simulink model "combinedTxRx_ADIDMA"  (R2017b)
settings: Solver=FixedStepDiscrete  StartTime=0.0  StopTime=10.0  RelTol=1e-3
InitFcn:
  | numHeaderBits = 16;
  | %numPreambleBits = 250;
  | AGCBarkerSymbols = 160+28;
  | EQTrainingSymbols = 250;
  | CRCGeneratorLag = 34; % CRCLen + 2
  | 
  | %% AGC Preamble
  | B13bipolar = [0 0 0 0 0 2 2 0 0 2 0 2];
  | rep = [B13bipolar, B13bipolar(1:4)];
  | AGCBarker = repmat(rep,1,10);
  | % Second preamble part
  | B11bipolar = [0 0 0 2 2 2 0 2  2 0 2];
  | TimingBarker = [B11bipolar,B11bipolar,B11bipolar,B11bipolar(1:6)];
  | PreambleBarkersInts = [AGCBarker, TimingBarker];
  | % Convert integer into their bit representation
  | PreambleBarkersBits = zeros(1,length(PreambleBarkersInts)*2);
  | PreambleBarkersBits(1:2:end) = (PreambleBarkersInts==2);
  | 
  | % Constants
  | % First preamble part
  | B13bipolar = [0 0 0 0 0 2 2 0 0 2 0 2];
  | rep = [B13bipolar, B13bipolar(1:4)];
  | AGCBarker = repmat(rep,1,10);
  | % Second preamble part
  | B11bipolar = [0 0 0 2 2 2 0 2  2 0 2];
  | TimingBarker = [B11bipolar,B11bipolar,B11bipolar(1:6)];
  | PreambleBarkersInts = [AGCBarker, TimingBarker];
  | % Convert integer into their bit representation
  | PreambleBarkersBits = false(1,length(PreambleBarkersInts)*2);
  | PreambleBarkersBits(1:2:end) = logical(PreambleBarkersInts==2);
  | pLen = uint16(length(PreambleBarkersBits));
  | 
  | 
  | %%%%%%%%%%%%%%%%%%%%%%%%%%
  | %% RX
  | %%%%%%%%%%%%%%%%%%%%%%%%%%
  | 
  | barker = comm.BarkerCode('SamplesPerFrame', 28, 'Length', 11);
  | seq = barker()+1;
  | M = 4;
  | hPSKModTrain   = comm.PSKModulator(M, ...
  |     'PhaseOffset',pi/4, ...
  |     'SymbolMapping','Binary');
  | xPreambleSeq = hPSKModTrain(seq);
  | 
  | 
  | %%%%%%%%%%%%
  | 
  | % AGC Preamble
  | reps = 5;
  | barker = comm.BarkerCode('SamplesPerFrame', 16, 'Length', 13);
  | seq = barker()+1;
  | %preamble = zeros(16*reps,1);
  | preambleFull = repmat(seq,reps,1);
  | rctFilt = comm.RaisedCosineTransmitFilter('FilterSpanInSymbols', 128,...
  | 'RolloffFactor',0.5,...
  | 'OutputSamplesPerSymbol',4);
  | preambleFullFilt = rctFilt(preambleFull);
  | 
  | %%%%%%%%%%%%
  | 
  | RadioSampleRate = 1e6;
  | %RadioSampleRate = 20e6;
  | RadioFrameLength = 1e5;
  | 
  | VibertiTracebackLength = 34+20;
  | numTrainingSamples = 250;
  | crc32Poly = [1 0 0 0 0 0 1 0 0 1 1 0 0 0 0 0 1 0 0 0 1 1 1 0 1 1 0 1 1 0 1 1 1];
  | crcDecodeLag = length(crc32Poly)-1+2;
  | 
  | %%%%%%%%%%%%
  | 
  | beta = 0.5;
  | span = 8;
  | sps = 4;
  | filterGain = 1;
  | coeff = rcosdesign(beta, span, sps, 'sqrt')*filterGain;
  | 
  | %%%%%%%%%%%%
  | 
  | samplesPerSymbol = 4;
  | maxPacketBits = 8*1500;
  | bItsPerSymbol = 2;
  | CodeRate = 2;
  | tailSymbols = 40;
  | maxPayloadSymbols = maxPacketBits*CodeRate/bItsPerSymbol+tailSymbols;
  | 
  | 
  | %%%%%%%%%%%%
  | 
  | NormalizedLoopBandwidths = 0.01:0.01:0.4;
  | K1 = zeros(length(NormalizedLoopBandwidths),1);
  | K2 = zeros(length(NormalizedLoopBandwidths),1);
  | 
  | for index=1:length(NormalizedLoopBandwidths)
  |     DampingFactor = 4*1/sqrt(2);
  |     samplesPerSymbolFR = 1;
  |     NormalizedLoopBandwidth = NormalizedLoopBandwidths(index);
  | 
  |     %%
  |     PhaseRecoveryLoopBandwidth = NormalizedLoopBandwidth*samplesPerSymbolFR;
  | 
  |     PhaseRecoveryGain = samplesPerSymbolFR;
  | 
  |     PhaseErrorDetectorGain = 1;
  | 
  |     %%
  |     theta = PhaseRecoveryLoopBandwidth/...
  |         ((DampingFactor + 0.25/DampingFactor)*samplesPerSymbolFR);
  | 
  |     d = 1 + 2*DampingFactor*theta + theta*theta;
  | 
  |     % K1
  |     K1(index) = (4*DampingFactor*theta/d)/...
  |         (PhaseErrorDetectorGain*PhaseRecoveryGain);
  |     % K2
  |     K2(index) = (4/samplesPerSymbol*theta*theta/d)/...
  |         (PhaseErrorDetectorGain*PhaseRecoveryGain);
  | 
  | end
  | K1 = fi(K1,0);
  | K2 = fi(K2,0);
undefined symbols (not defined in the file or in its folder): j
libraries: simulink x20, dsphdlfiltering x20, hdlsllib x7, dspsigops x4, commseqgen3 x3, commdigbbndpm3 x3, commcrc2 x2, commcnvcod2 x2, commfilt2 x2, commsource2 x1, dspstat3 x1
(part 1 of 3)
settings Model: Creator=tcollins  LastModifiedBy=tcollins
settings OptimizationCC: BlockReduction=off  ConditionallyExecuteInputs=off  DefaultParameterBehavior=Inlined
settings DebuggingCC: AlgebraicLoopMsg=error  SingleTaskRateTransMsg=error
settings HardwareCC: ProdBitPerPointer=32  ProdBitPerSizeT=32  ProdBitPerPtrDiffT=32  ProdLargestAtomicFloat=None  ProdIntDivRoundTo=Undefined  ProdEndianess=Unspecified  ProdWordSize=32  ProdHWDeviceType=ASIC/FPGA->ASIC/FPGA  ProdEqTarget=off
settings CodeAppCC: StateflowObjectComments=on

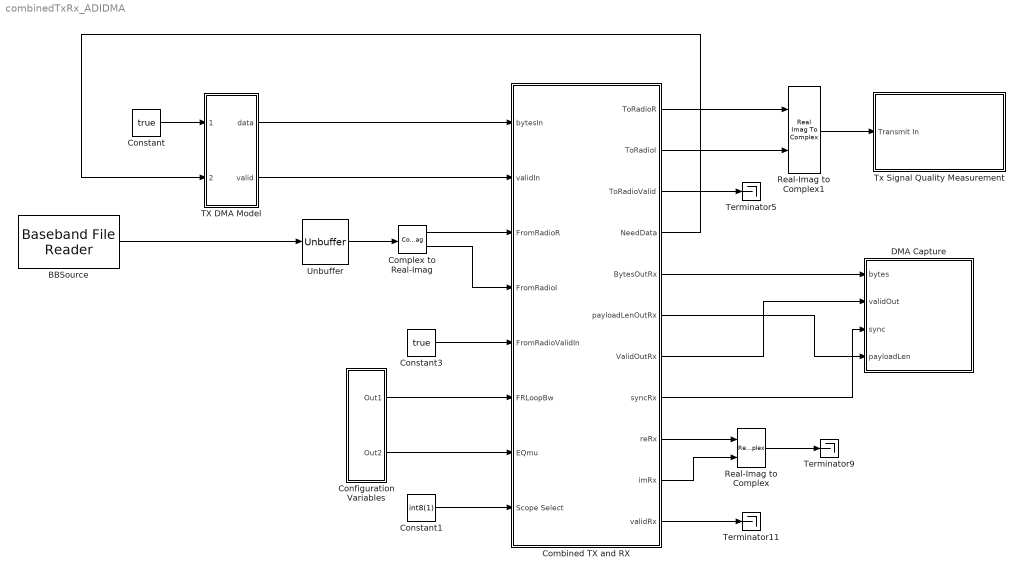
== system combinedTxRx_ADIDMA ==
  BBSource : commsource2/Baseband File Reader  Filename=PlutoCaptureQPSK.bb  InheritSampleTimeFromFile=off  SampleTime=100000/(RadioSampleRate)  SamplesPerFrame=100000  CyclicRepetition=off  FileEndOutputPort=off  SimulateUsing=Interpreted execution
      settings: SourceProductName=Communications System Toolbox  SourceProductBaseCode=CM
  Combined TX and RX : Subsystem  TreatAsAtomicUnit=on
  Complex to Real-Imag : ComplexToRealImag
  Configuration Variables : Subsystem
  Constant : Constant  Value=true  SampleTime=-1
  Constant1 : Constant  Value=int8(1)  SampleTime=1/RadioSampleRate
  Constant3 : Constant  Value=true  SampleTime=1/RadioSampleRate
  DMA Capture : MATLAB Function  TreatAsAtomicUnit=on
  Real-Imag to Complex : RealImagToComplex
  Real-Imag to Complex1 : RealImagToComplex
  TX DMA Model : Subsystem
  Terminator11 : Terminator
  Terminator5 : Terminator
  Terminator9 : Terminator
  Tx Signal Quality Measurement : Subsystem
  Unbuffer : Unbuffer
  wires:
  Real-Imag to Complex/1 -> Terminator9/1
  BBSource/1 -> Unbuffer/1
  Unbuffer/1 -> Complex to Real-Imag/1
  Complex to Real-Imag/1 -> Combined TX and RX/3(FromRadioR)
  Complex to Real-Imag/2 -> Combined TX and RX/4(FromRadioI)
  Constant3/1 -> Combined TX and RX/5(FromRadioValidIn)
  Combined TX and RX/1(ToRadioR) -> Real-Imag to Complex1/1
  Combined TX and RX/2(ToRadioI) -> Real-Imag to Complex1/2
  Combined TX and RX/3(ToRadioValid) -> Terminator5/1
  Combined TX and RX/5(BytesOutRx) -> DMA Capture/1(bytes)
  Combined TX and RX/6(payloadLenOutRx) -> DMA Capture/4(payloadLen)
  Combined TX and RX/8(syncRx) -> DMA Capture/3(sync)
  Combined TX and RX/9(reRx) -> Real-Imag to Complex/1
  Combined TX and RX/10(imRx) -> Real-Imag to Complex/2
  Combined TX and RX/11(validRx) -> Terminator11/1
  Real-Imag to Complex1/1 -> Tx Signal Quality Measurement/1(Transmit In)
  Constant1/1 -> Combined TX and RX/8(Scope Select)
  Configuration Variables/1(Out1) -> Combined TX and RX/6(FRLoopBw)
  Configuration Variables/2(Out2) -> Combined TX and RX/7(EQmu)
  Combined TX and RX/7(ValidOutRx) -> DMA Capture/2(validOut)
  Constant/1 -> TX DMA Model/1(enable)
  Combined TX and RX/4(NeedData) -> TX DMA Model/2(enableTx)
  TX DMA Model/1(data) -> Combined TX and RX/1(bytesIn)
  TX DMA Model/2(valid) -> Combined TX and RX/2(validIn)

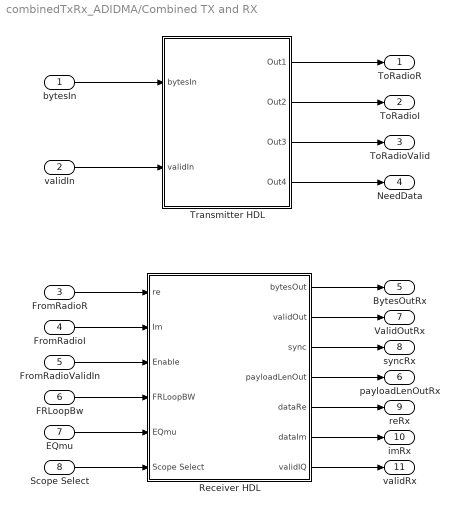
== system combinedTxRx_ADIDMA/Combined TX and RX ==
  bytesIn : Inport
  validIn : Inport  Port=2
  FromRadioR : Inport  Port=3
  FromRadioI : Inport  Port=4
  FromRadioValidIn : Inport  Port=5
  FRLoopBw : Inport  Port=6
  EQmu : Inport  Port=7
  Scope Select : Inport  Port=8
  Receiver HDL : Subsystem  TreatAsAtomicUnit=on
      mask Display: image('/home/tcollins/Downloads/Analog_Devices_Logo3.svg');
  Transmitter HDL : Subsystem  TreatAsAtomicUnit=on
      mask Display: image('/home/tcollins/Downloads/Analog_Devices_Logo3.svg');
  ToRadioR : Outport
  ToRadioI : Outport  Port=2
  ToRadioValid : Outport  Port=3
  NeedData : Outport  Port=4
  BytesOutRx : Outport  Port=5
  payloadLenOutRx : Outport  Port=6
  ValidOutRx : Outport  Port=7
  syncRx : Outport  Port=8
  reRx : Outport  Port=9
  imRx : Outport  Port=10
  validRx : Outport  Port=11
  wires:
  Receiver HDL/2(validOut) -> ValidOutRx/1
  Receiver HDL/6(dataIm) -> imRx/1
  Receiver HDL/3(sync) -> syncRx/1
  Receiver HDL/4(payloadLenOut) -> payloadLenOutRx/1
  Receiver HDL/7(validIQ) -> validRx/1
  Receiver HDL/5(dataRe) -> reRx/1
  Receiver HDL/1(bytesOut) -> BytesOutRx/1
  validIn/1 -> Transmitter HDL/2("validIn ")
  Transmitter HDL/2(Out2) -> ToRadioI/1
  Transmitter HDL/3(Out3) -> ToRadioValid/1
  Transmitter HDL/1(Out1) -> ToRadioR/1
  bytesIn/1 -> Transmitter HDL/1(bytesIn)
  Transmitter HDL/4(Out4) -> NeedData/1
  FromRadioR/1 -> Receiver HDL/1(re)
  FromRadioI/1 -> Receiver HDL/2(Im)
  FromRadioValidIn/1 -> Receiver HDL/3(Enable)
  FRLoopBw/1 -> Receiver HDL/4(FRLoopBW)
  EQmu/1 -> Receiver HDL/5(EQmu)
  Scope Select/1 -> Receiver HDL/6(Scope Select)

== system combinedTxRx_ADIDMA/Configuration Variables ==
  1/mu : Constant  Value=1000  OutDataTypeStr=int16  SampleTime=-1
  Index of LBW Lookup : Constant  Value=int16(10)  SampleTime=1/RadioSampleRate
  Out1 : Outport
  Out2 : Outport  Port=2
  wires:
  1/mu/1 -> Out2/1
  Index of LBW Lookup/1 -> Out1/1

== system combinedTxRx_ADIDMA/TX DMA Model ==
  note: Keep On
  enable : Inport
  enableTx : Inport  Port=2
  DMA Model Driver : MATLAB Function  TreatAsAtomicUnit=on
  Data Type Conversion : DataTypeConversion  OutDataTypeStr=fixdt(0,64,0)
  Delay : Delay  DelayLength=1
  Downsample1 : DownSample  N=4  RateOptions=Allow multirate processing
  Downsample2 : DownSample  N=4  RateOptions=Allow multirate processing
  Logical Operator : Logic  Operator=OR  AllPortsSameDT=off  OutDataTypeStr=boolean
  Logical Operator1 : Logic  Operator=NOT  AllPortsSameDT=off  OutDataTypeStr=boolean
  Repeat : dspsigops/Repeat  N=4  InputProcessing=Columns as channels (frame based)  RateOptions=Allow multirate processing  ic=0  mode=Unused parameter value
      settings: SourceProductName=DSP System Toolbox
  Repeat1 : dspsigops/Repeat  N=4  InputProcessing=Columns as channels (frame based)  RateOptions=Allow multirate processing  ic=0  mode=Unused parameter value
      settings: SourceProductName=DSP System Toolbox
  Signal Specification1 : SignalSpecification  OutDataTypeStr=boolean  SampleTime=1e-6
  data : Outport
  valid : Outport  Port=2
  wires:
  Downsample2/1 -> Logical Operator/1, Logical Operator1/1
  Logical Operator/1 -> DMA Model Driver/1(driver)
  Repeat1/1 -> valid/1
  DMA Model Driver/2(valid) -> Repeat1/1
  enableTx/1 -> Downsample1/1
  Data Type Conversion/1 -> Repeat/1
  Downsample1/1 -> Delay/1
  Signal Specification1/1 -> Downsample2/1
  Delay/1 -> DMA Model Driver/2(enable)
  Logical Operator1/1 -> Logical Operator/2
  DMA Model Driver/1(payload) -> Data Type Conversion/1
  enable/1 -> Signal Specification1/1
  Repeat/1 -> data/1

== system combinedTxRx_ADIDMA/Tx Signal Quality Measurement ==
  Transmit In : Inport
  Constellation Diagram : ConstellationDiagram
  Raised Cosine Receive Filter : commfilt2/Raised Cosine Receive Filter  filtType=Square root  R=0.5  filtSpan=8  N=4  downFactor=4  downOffset=0  filterGain=1  RateOptions=Allow multirate processing  framing=Mute  checkCoeff=off  variableName=rcRxFilt  currentFiltSpan=8  D=(8)/2  inputOffset=0  sampMode=Mute  saveAsFlag=0  rateMode=Downsampling  checkGain=Normalized  launchFVT=on  roundingMode=Floor  overflowMode=off  coeffDataTypeStr=Inherit: Same word length as input  coeffMin=[]  coeffMax=[]  coeffLastDataTypeStr=Inherit: Same word length as input  accumDataTypeStr=Inherit: Same as product output  accumLastDataTypeStr=Inherit: Same as product output  outputDataTypeStr=Inherit: Same as accumulator  outputMin=[]  outputMax=[]  outputLastDataTypeStr=Inherit: Same as accumulator
  wires:
  Transmit In/1 -> Raised Cosine Receive Filter/1
  Raised Cosine Receive Filter/1 -> Constellation Diagram/1  "Measured"

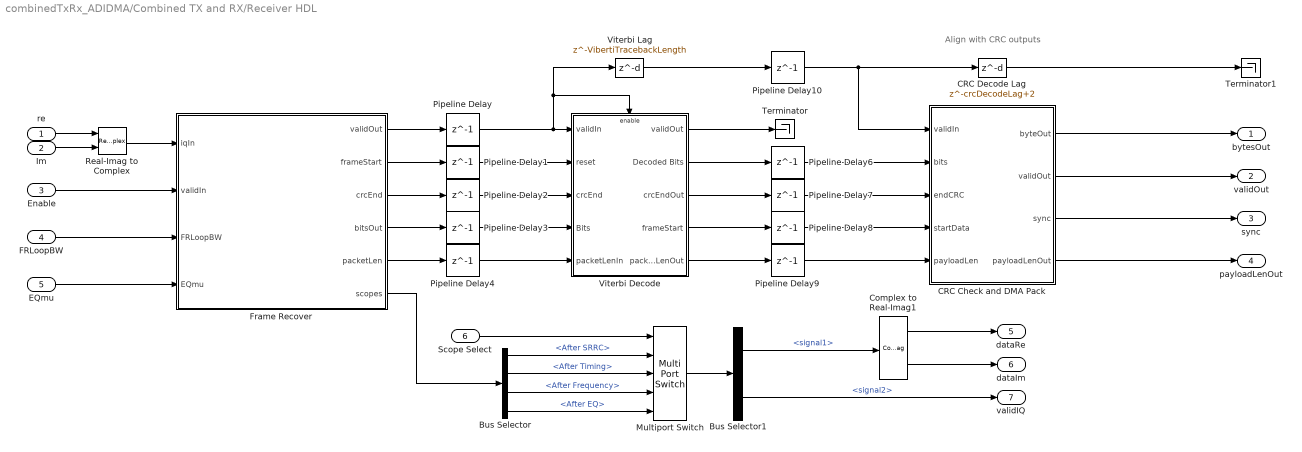
== system combinedTxRx_ADIDMA/Combined TX and RX/Receiver HDL ==
  note: Align with CRC outputs
  re : Inport  OutDataTypeStr=int16
  Im : Inport  Port=2  OutDataTypeStr=int16
  Enable : Inport  Port=3
  FRLoopBW : Inport  Port=4
  EQmu : Inport  Port=5
  Scope Select : Inport  Port=6
  Bus Selector : BusSelector  OutputSignals=After SRRC,After Timing,After Frequency,After EQ
  Bus Selector1 : BusSelector  OutputSignals=signal1,signal2
  CRC Check and DMA Pack : Subsystem
  CRC Decode Lag : Delay  DelayLength=crcDecodeLag+2
  Complex to Real-Imag1 : ComplexToRealImag
  Frame Recover : Subsystem
  Multiport Switch : MultiPortSwitch  Inputs=4
  Pipeline Delay{,1..4,6..10} (10 alike) : Delay  DelayLength=1
  Real-Imag to Complex : RealImagToComplex
  Terminator : Terminator
  Terminator1 : Terminator
  Viterbi Decode : Subsystem  TreatAsAtomicUnit=on
  Viterbi Lag : Delay  DelayLength=VibertiTracebackLength
  bytesOut : Outport
  validOut : Outport  Port=2
  sync : Outport  Port=3
  payloadLenOut : Outport  Port=4
  dataRe : Outport  Port=5
  dataIm : Outport  Port=6
  validIQ : Outport  Port=7
  wires:
  re/1 -> Real-Imag to Complex/1
  Im/1 -> Real-Imag to Complex/2
  Complex to Real-Imag1/2 -> dataIm/1
  Complex to Real-Imag1/1 -> dataRe/1
  Frame Recover/5(packetLen) -> Pipeline Delay4/1
  Frame Recover/1(validOut) -> Pipeline Delay/1
  Real-Imag to Complex/1 -> Frame Recover/1(iqIn)
  Enable/1 -> Frame Recover/2(validIn)
  Frame Recover/2(frameStart) -> Pipeline Delay1/1
  Frame Recover/3(crcEnd) -> Pipeline Delay2/1
  Frame Recover/4(bitsOut) -> Pipeline Delay3/1
  Viterbi Decode/3(crcEndOut) -> Pipeline Delay7/1
  Viterbi Decode/4(frameStart) -> Pipeline Delay8/1
  Viterbi Decode/5(packetLenOut) -> Pipeline Delay9/1
  CRC Check and DMA Pack/1(byteOut) -> bytesOut/1
  CRC Check and DMA Pack/2(validOut) -> validOut/1
  Pipeline Delay1/1 -> Viterbi Decode/2(reset)
  Pipeline Delay3/1 -> Viterbi Decode/4(Bits)
  Pipeline Delay4/1 -> Viterbi Decode/5(packetLenIn)
  Pipeline Delay8/1 -> CRC Check and DMA Pack/4(startData)
  Pipeline Delay6/1 -> CRC Check and DMA Pack/2(bits)
  Pipeline Delay9/1 -> CRC Check and DMA Pack/5(payloadLen)
  Pipeline Delay7/1 -> CRC Check and DMA Pack/3(endCRC)
  CRC Check and DMA Pack/3(sync) -> sync/1
  Pipeline Delay2/1 -> Viterbi Decode/3(crcEnd)
  Viterbi Decode/2(Decoded Bits) -> Pipeline Delay6/1
  Pipeline Delay10/1 -> CRC Check and DMA Pack/1(validIn), CRC Decode Lag/1
  CRC Check and DMA Pack/4(payloadLenOut) -> payloadLenOut/1
  Pipeline Delay/1 -> Viterbi Decode/Enable, Viterbi Lag/1, Viterbi Decode/1(validIn)
  Viterbi Decode/1(validOut) -> Terminator/1
  Viterbi Lag/1 -> Pipeline Delay10/1
  CRC Decode Lag/1 -> Terminator1/1
  FRLoopBW/1 -> Frame Recover/3(FRLoopBW)
  EQmu/1 -> Frame Recover/4(EQmu)
  Frame Recover/6(scopes) -> Bus Selector/1
  Bus Selector/1 -> Multiport Switch/2  "<After SRRC>"
  Bus Selector/3 -> Multiport Switch/4  "<After Frequency>"
  Bus Selector/2 -> Multiport Switch/3  "<After Timing>"
  Scope Select/1 -> Multiport Switch/1
  Multiport Switch/1 -> Bus Selector1/1
  Bus Selector/4 -> Multiport Switch/5  "<After EQ>"
  Bus Selector1/1 -> Complex to Real-Imag1/1  "<signal1>"
  Bus Selector1/2 -> validIQ/1  "<signal2>"

== system combinedTxRx_ADIDMA/Combined TX and RX/Transmitter HDL ==
  bytesIn : Inport
  "validIn " : Inport  Port=2
  Transmitter HDL : Subsystem  TreatAsAtomicUnit=on
  Out1 : Outport
  Out2 : Outport  Port=2
  Out3 : Outport  Port=3
  Out4 : Outport  Port=4
  wires:
  Transmitter HDL/4(Need Data) -> Out4/1
  Transmitter HDL/2(imag) -> Out2/1
  Transmitter HDL/1(real) -> Out1/1
  Transmitter HDL/3(validOut) -> Out3/1
  bytesIn/1 -> Transmitter HDL/1(bytesIn)
  "validIn "/1 -> Transmitter HDL/2(validIn)

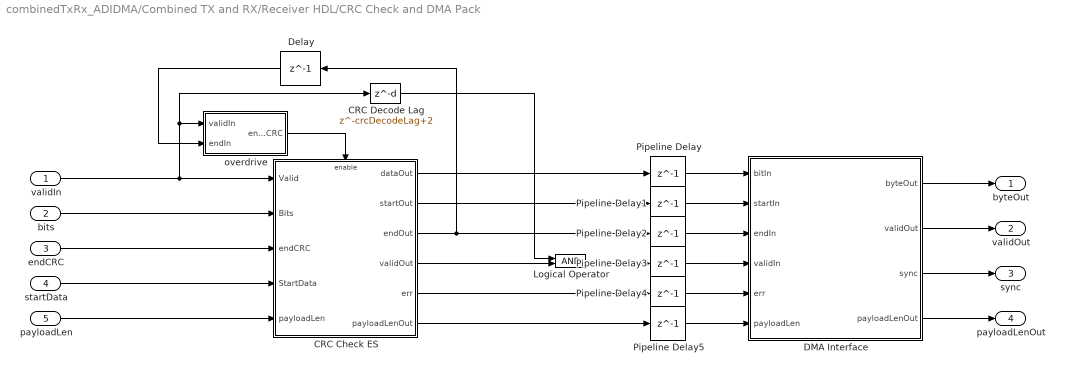
== system combinedTxRx_ADIDMA/Combined TX and RX/Receiver HDL/CRC Check and DMA Pack ==
  validIn : Inport
  bits : Inport  Port=2
  endCRC : Inport  Port=3
  startData : Inport  Port=4
  payloadLen : Inport  Port=5
  CRC Check ES : Subsystem
  CRC Decode Lag : Delay  DelayLength=crcDecodeLag+2
  DMA Interface : Subsystem
  Delay : Delay  DelayLength=1
  Logical Operator : Logic  AllPortsSameDT=off  OutDataTypeStr=boolean
  Pipeline Delay{,1..5} (6 alike) : Delay  DelayLength=1
  overdrive : MATLAB Function  TreatAsAtomicUnit=on
  byteOut : Outport
  validOut : Outport  Port=2
  sync : Outport  Port=3
  payloadLenOut : Outport  Port=4
  wires:
  DMA Interface/2(validOut) -> validOut/1
  CRC Check ES/3(endOut) -> Delay/1, Pipeline Delay2/1
  DMA Interface/1(byteOut) -> byteOut/1
  CRC Check ES/2(startOut) -> Pipeline Delay1/1
  CRC Check ES/1(dataOut) -> Pipeline Delay/1
  CRC Check ES/5(err) -> Pipeline Delay4/1
  bits/1 -> CRC Check ES/2(Bits)
  DMA Interface/3(sync) -> sync/1
  payloadLen/1 -> CRC Check ES/5(payloadLen)
  startData/1 -> CRC Check ES/4(StartData)
  CRC Check ES/6(payloadLenOut) -> Pipeline Delay5/1
  endCRC/1 -> CRC Check ES/3(endCRC)
  Pipeline Delay/1 -> DMA Interface/1(bitIn)
  Pipeline Delay1/1 -> DMA Interface/2(startIn)
  Pipeline Delay2/1 -> DMA Interface/3(endIn)
  Pipeline Delay3/1 -> DMA Interface/4(validIn)
  Pipeline Delay4/1 -> DMA Interface/5(err)
  Pipeline Delay5/1 -> DMA Interface/6(payloadLen)
  CRC Decode Lag/1 -> Logical Operator/1
  CRC Check ES/4(validOut) -> Logical Operator/2
  validIn/1 -> CRC Check ES/1(Valid), CRC Decode Lag/1, overdrive/1(validIn)
  Delay/1 -> overdrive/2(endIn)
  DMA Interface/4(payloadLenOut) -> payloadLenOut/1
  Logical Operator/1 -> Pipeline Delay3/1
  overdrive/1(enableCRC) -> CRC Check ES/Enable

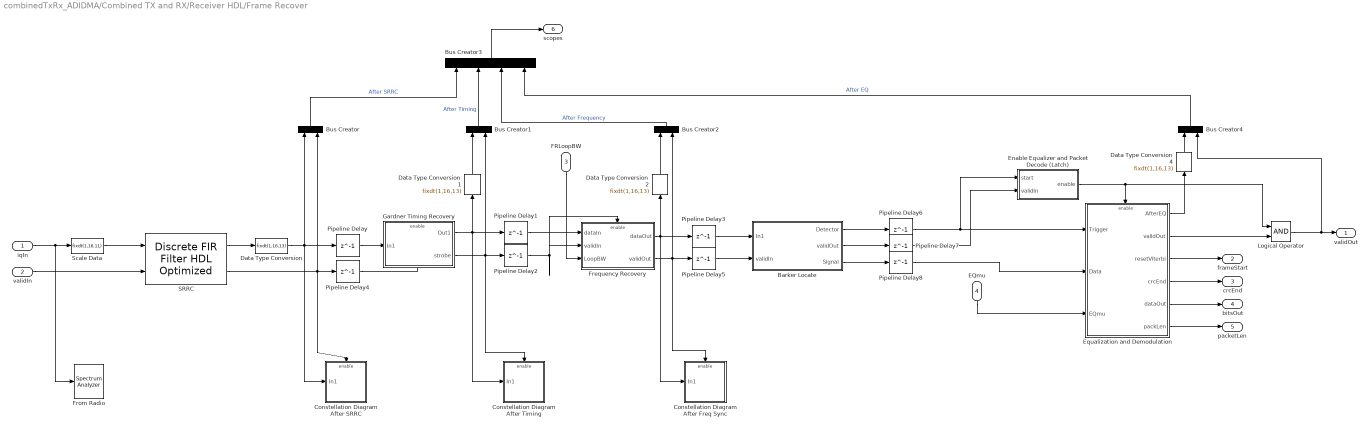
== system combinedTxRx_ADIDMA/Combined TX and RX/Receiver HDL/Frame Recover ==
  iqIn : Inport
  validIn : Inport  Port=2
  FRLoopBW : Inport  Port=3
  EQmu : Inport  Port=4
  Barker Locate : Subsystem  mask{Threshold=1}
  Bus Creator{,1..2,4} (4 alike) : BusCreator  Inputs=2
  Bus Creator3 : BusCreator  Inputs=4
  Constellation Diagram After Freq Sync : Subsystem
  Constellation Diagram After SRRC : Subsystem
  Constellation Diagram After Timing : Subsystem
  Data Type Conversion{,1..2,4} (4 alike) : DataTypeConversion  OutDataTypeStr=fixdt(1,16,13)
  Enable Equalizer and Packet Decode (Latch) : MATLAB Function  TreatAsAtomicUnit=on
  Equalization and Demodulation : Subsystem
  Frequency Recovery : Subsystem
  From Radio : SpectrumAnalyzer
  Gardner Timing Recovery : Subsystem
  Logical Operator : Logic  AllPortsSameDT=off  OutDataTypeStr=boolean
  Pipeline Delay{,1..8} (9 alike) : Delay  DelayLength=1
  SRRC : dsphdlfiltering/Discrete FIR Filter HDL Optimized  Numerator=coeff  Sharing=off  SharingFactor=2  SimulateUsing=Code generation  roundingMode=Floor  overflowMode=on  CoefficientsDataTypeStr=Inherit: Same word length as input  CoefficientsMin=[]  CoefficientsMax=[]  OutputDataTypeStr=fixdt(1,16,11)  OutputMin=[]  OutputMax=[]  ValidInPort=on  ReadyPort=off
      settings: SourceProductName=DSP System Toolbox  SourceProductBaseCode=DS
  Scale Data : DataTypeConversion  OutDataTypeStr=fixdt(1,16,11)  ConvertRealWorld=Stored Integer (SI)  SaturateOnIntegerOverflow=on
  validOut : Outport
  frameStart : Outport  Port=2
  crcEnd : Outport  Port=3
  bitsOut : Outport  Port=4
  packetLen : Outport  Port=5
  scopes : Outport  Port=6
  wires:
  Equalization and Demodulation/3(resetViterbi) -> frameStart/1
  Barker Locate/2(validOut) -> Pipeline Delay7/1
  Equalization and Demodulation/4(crcEnd) -> crcEnd/1
  Enable Equalizer and Packet Decode (Latch)/1(enable) -> Logical Operator/1, Equalization and Demodulation/Enable
  Equalization and Demodulation/5(dataOut) -> bitsOut/1
  SRRC/2 -> Pipeline Delay4/1, Constellation Diagram After SRRC/Enable, Bus Creator/2
  SRRC/1 -> Data Type Conversion/1
  iqIn/1 -> From Radio/1, Scale Data/1
  validIn/1 -> SRRC/2
  Barker Locate/3(Signal) -> Pipeline Delay8/1
  Equalization and Demodulation/2(validOut) -> Logical Operator/2
  Scale Data/1 -> SRRC/1
  Equalization and Demodulation/6(packLen) -> packetLen/1
  Barker Locate/1(Detector) -> Pipeline Delay6/1
  Equalization and Demodulation/1(AfterEQ) -> Data Type Conversion4/1
  Pipeline Delay1/1 -> Frequency Recovery/1(dataIn)
  Pipeline Delay2/1 -> Frequency Recovery/2(validIn), Frequency Recovery/Enable
  Pipeline Delay3/1 -> Barker Locate/1(In1)
  Pipeline Delay5/1 -> Barker Locate/2(validIn)
  Pipeline Delay6/1 -> Enable Equalizer and Packet Decode (Latch)/1(start), Equalization and Demodulation/1(Trigger)
  Pipeline Delay7/1 -> Enable Equalizer and Packet Decode (Latch)/2(validIn)
  Pipeline Delay8/1 -> Equalization and Demodulation/2(Data)
  Logical Operator/1 -> Bus Creator4/2, validOut/1
  Data Type Conversion/1 -> Pipeline Delay/1, Constellation Diagram After SRRC/1(In1), Bus Creator/1
  Pipeline Delay/1 -> Gardner Timing Recovery/1(In1)
  Pipeline Delay4/1 -> Gardner Timing Recovery/Enable
  FRLoopBW/1 -> Frequency Recovery/3(LoopBW)
  EQmu/1 -> Equalization and Demodulation/3(EQmu)
  Gardner Timing Recovery/2(strobe) -> Constellation Diagram After Timing/Enable, Bus Creator1/2, Pipeline Delay2/1
  Gardner Timing Recovery/1(Out1) -> Constellation Diagram After Timing/1(In1), Data Type Conversion1/1, Pipeline Delay1/1
  Frequency Recovery/1(dataOut) -> Pipeline Delay3/1, Constellation Diagram After Freq Sync/1(In1), Data Type Conversion2/1
  Frequency Recovery/2(validOut) -> Pipeline Delay5/1, Constellation Diagram After Freq Sync/Enable, Bus Creator2/2
  Bus Creator/1 -> Bus Creator3/1  "After SRRC"
  Bus Creator1/1 -> Bus Creator3/2  "After Timing"
  Bus Creator2/1 -> Bus Creator3/3  "After Frequency"
  Bus Creator3/1 -> scopes/1
  Bus Creator4/1 -> Bus Creator3/4  "After EQ"
  Data Type Conversion1/1 -> Bus Creator1/1
  Data Type Conversion2/1 -> Bus Creator2/1
  Data Type Conversion4/1 -> Bus Creator4/1

== system combinedTxRx_ADIDMA/Combined TX and RX/Receiver HDL/Viterbi Decode ==
  validIn : Inport
  reset : Inport  Port=2
  crcEnd : Inport  Port=3
  Bits : Inport  Port=4
  packetLenIn : Inport  Port=5
  Enable : EnablePort
  Delay : Delay  DelayLength=1
  "Pipeline Delay (REMOVE BEFORE SYNTH, ONLY FOR SIMULATION)" : Delay  Commented=on  DelayLength=20
  Viterbi Decoder : commcnvcod2/Viterbi Decoder  trellis=poly2trellis(7, [171 133])  isPunctured=off  punctureVector=[1; 1; 0; 1; 0; 1]  erasures=off  dectype=Hard decision  nsdecb=4  runSigValErrCheck=off  tbdepth=VibertiTracebackLength-20  opmode=Continuous  reset=on  delayedResetAction=on  smWordLength=16  outDataType=boolean
      settings: SourceProductName=Communications System Toolbox  SourceProductBaseCode=CM
  Viterbi Lag{,1..3} (4 alike) : Delay  DelayLength=VibertiTracebackLength
  validOut : Outport  InitialOutput=0
  Decoded Bits : Outport  Port=2  InitialOutput=0
  crcEndOut : Outport  Port=3  InitialOutput=0
  frameStart : Outport  Port=4  InitialOutput=0
  packetLenOut : Outport  Port=5  InitialOutput=0
  wires:
  reset/1 -> Viterbi Lag2/1, Viterbi Decoder/2
  Bits/1 -> Viterbi Decoder/1
  validIn/1 -> Viterbi Lag/1
  Viterbi Lag3/1 -> packetLenOut/1
  Viterbi Lag2/1 -> Delay/1
  Viterbi Lag1/1 -> crcEndOut/1
  Viterbi Lag/1 -> validOut/1
  packetLenIn/1 -> Viterbi Lag3/1
  crcEnd/1 -> Viterbi Lag1/1
  Delay/1 -> frameStart/1
  Viterbi Decoder/1 -> Decoded Bits/1

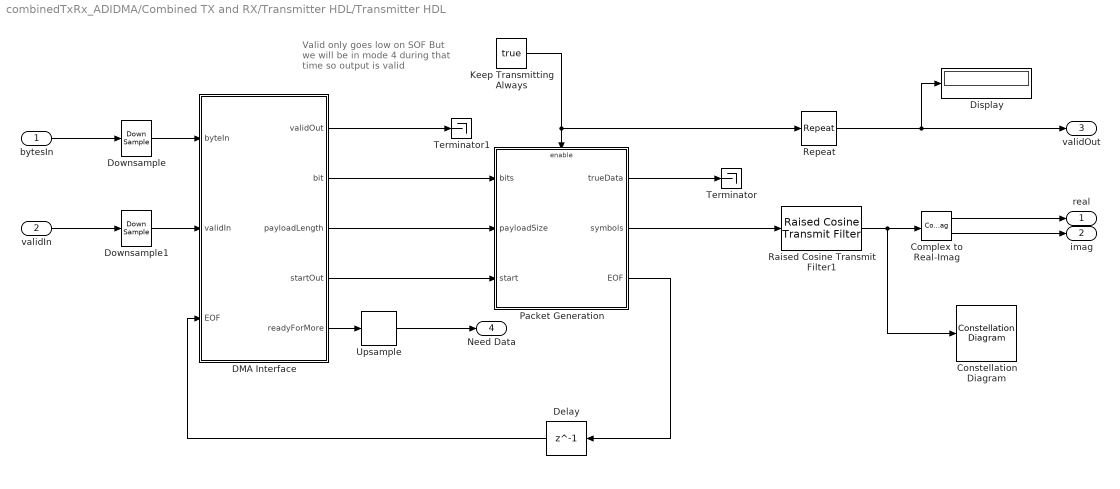
== system combinedTxRx_ADIDMA/Combined TX and RX/Transmitter HDL/Transmitter HDL ==
  note: Valid only goes low on SOF
      | But we will be in mode 4 during
      | that time so output is valid
  bytesIn : Inport
  validIn : Inport  Port=2
  Complex to Real-Imag : ComplexToRealImag
  Constellation Diagram : ConstellationDiagram
  DMA Interface : Subsystem
  Delay : Delay  DelayLength=1
  Display : Display
  Downsample : DownSample  N=4  RateOptions=Allow multirate processing
  Downsample1 : DownSample  N=4  RateOptions=Allow multirate processing
  Keep Transmitting Always : Constant  Value=true  SampleTime=-1
  Packet Generation : Subsystem
  Raised Cosine Transmit Filter1 : commfilt2/Raised Cosine Transmit Filter  filtType=Square root  R=0.5  filtSpan=8  N=4  filterGain=1  RateOptions=Allow multirate processing  framing=Mute  checkCoeff=off  variableName=rcTxFilt1  checkGain=Normalized  sampMode=Mute  saveAsFlag=0  currentFiltSpan=8  D=(8)/2  launchFVT=on  roundingMode=Floor  overflowMode=off  coeffDataTypeStr=Inherit: Same word length as input  coeffMin=[]  coeffMax=[]  coeffLastDataTypeStr=Inherit: Same word length as input  outputMode=Binary point scaling  outputWordLength=16  outputFracLength=14  outputDataTypeStr=fixdt(1,16,14)  outputMin=[]  outputMax=[]  outputLastDataTypeStr=fixdt(1,16,14)
  Repeat : dspsigops/Repeat  N=4  InputProcessing=Columns as channels (frame based)  RateOptions=Allow multirate processing  ic=0  mode=Unused parameter value
      settings: SourceProductName=DSP System Toolbox
  Terminator : Terminator
  Terminator1 : Terminator
  Upsample : dspsigops/Upsample  N=4  phase=0  RateOptions=Allow multirate processing  ic=0  mode=Unused parameter value
  real : Outport
  imag : Outport  Port=2
  validOut : Outport  Port=3
  Need Data : Outport  Port=4
  wires:
  Raised Cosine Transmit Filter1/1 -> Constellation Diagram/1, Complex to Real-Imag/1
  Complex to Real-Imag/1 -> real/1
  Complex to Real-Imag/2 -> imag/1
  DMA Interface/2(bit) -> Packet Generation/1(bits)
  DMA Interface/3(payloadLength) -> Packet Generation/2(payloadSize)
  DMA Interface/4(startOut) -> Packet Generation/3(start)
  Packet Generation/2(symbols) -> Raised Cosine Transmit Filter1/1
  DMA Interface/5(readyForMore) -> Upsample/1
  Repeat/1 -> validOut/1, Display/1
  Packet Generation/1(trueData) -> Terminator/1
  Packet Generation/3(EOF) -> Delay/1
  Delay/1 -> DMA Interface/3(EOF)
  bytesIn/1 -> Downsample/1
  validIn/1 -> Downsample1/1
  Upsample/1 -> Need Data/1
  Downsample/1 -> DMA Interface/1(byteIn)
  Downsample1/1 -> DMA Interface/2(validIn)
  DMA Interface/1(validOut) -> Terminator1/1
  Keep Transmitting Always/1 -> Packet Generation/Enable, Repeat/1

== system combinedTxRx_ADIDMA/Combined TX and RX/Receiver HDL/CRC Check and DMA Pack/CRC Check ES ==
  note: NOTE:
      | 	The Valid signal must be latched during a packet, which is
      | 	a bug (2018a Fixed).  Therefore we must use the CRC block in an enabled
      | 	subsystem
  Valid : Inport
  Bits : Inport  Port=2
  endCRC : Inport  Port=3
  StartData : Inport  Port=4
  payloadLen : Inport  Port=5
  Enable : EnablePort
  CRC Decode Lag : Delay  DelayLength=crcDecodeLag
  Convert To fi : DataTypeConversion  OutDataTypeStr=fixdt(0,1,0)  SaturateOnIntegerOverflow=on
  DEBUG: CRC Input : MATLAB Function  Commented=on  TreatAsAtomicUnit=on
  DEBUG: Check CRC Result : MATLAB Function  Commented=on  TreatAsAtomicUnit=on
  General CRC Syndrom Detector HDL Optimized : commcrc2/General CRC Syndrome Detector HDL Optimized  Polynomial=crc32Poly  InitialState=0  DirectMethod=off  ReflectInput=off  ReflectCRCChecksum=off  FinalXORValue=0  SimulateUsing=Code generation
      settings: SourceProductName=Communications System Toolbox  SourceProductBaseCode=CM
  dataOut : Outport  InitialOutput=0
  startOut : Outport  Port=2  InitialOutput=0
  endOut : Outport  Port=3  InitialOutput=0
  validOut : Outport  Port=4  InitialOutput=0
  err : Outport  Port=5  InitialOutput=0
  payloadLenOut : Outport  Port=6  InitialOutput=0
  wires:
  Bits/1 -> Convert To fi/1, DEBUG: CRC Input/1(u)
  General CRC Syndrom Detector HDL Optimized/1 -> DEBUG: Check CRC Result/1(bits), dataOut/1
  General CRC Syndrom Detector HDL Optimized/3 -> DEBUG: Check CRC Result/3(done), endOut/1
  General CRC Syndrom Detector HDL Optimized/4 -> DEBUG: Check CRC Result/4(valid), validOut/1
  General CRC Syndrom Detector HDL Optimized/5 -> DEBUG: Check CRC Result/5(err), err/1
  General CRC Syndrom Detector HDL Optimized/2 -> DEBUG: Check CRC Result/2(start), startOut/1
  Convert To fi/1 -> General CRC Syndrom Detector HDL Optimized/1
  payloadLen/1 -> CRC Decode Lag/1
  CRC Decode Lag/1 -> payloadLenOut/1
  StartData/1 -> DEBUG: CRC Input/4(startFlag), General CRC Syndrom Detector HDL Optimized/2
  endCRC/1 -> DEBUG: CRC Input/3(endFlag), General CRC Syndrom Detector HDL Optimized/3
  Valid/1 -> General CRC Syndrom Detector HDL Optimized/4, DEBUG: CRC Input/2(enable)

== system combinedTxRx_ADIDMA/Combined TX and RX/Receiver HDL/CRC Check and DMA Pack/DMA Interface ==
  bitIn : Inport
  startIn : Inport  Port=2
  endIn : Inport  Port=3
  validIn : Inport  Port=4
  err : Inport  Port=5
  payloadLen : Inport  Port=6
  Bit Packer : MATLAB Function  TreatAsAtomicUnit=on
  Convert Payload Length To Bytes : Subsystem
  Data Type Conversion : DataTypeConversion  OutDataTypeStr=boolean
  Delay : Delay  DelayLength=1
  Delay Error To Last Byte of Out : Delay  DelayLength=1
  Display : Display
  byteOut : Outport
  validOut : Outport  Port=2
  sync : Outport  Port=3
  payloadLenOut : Outport  Port=4
  wires:
  bitIn/1 -> Data Type Conversion/1
  Delay/1 -> Bit Packer/3(endIn)
  Delay Error To Last Byte of Out/1 -> Bit Packer/4(err)
  Bit Packer/2(validOut) -> validOut/1
  Bit Packer/3(startOut) -> sync/1
  Bit Packer/1(byteOut) -> Display/1, byteOut/1
  err/1 -> Delay Error To Last Byte of Out/1
  validIn/1 -> Bit Packer/5(validIn)
  endIn/1 -> Delay/1
  startIn/1 -> Bit Packer/2(startIn)
  Data Type Conversion/1 -> Bit Packer/1(bitIn)
  payloadLen/1 -> Convert Payload Length To Bytes/1(In1)
  Convert Payload Length To Bytes/1(Out1) -> payloadLenOut/1

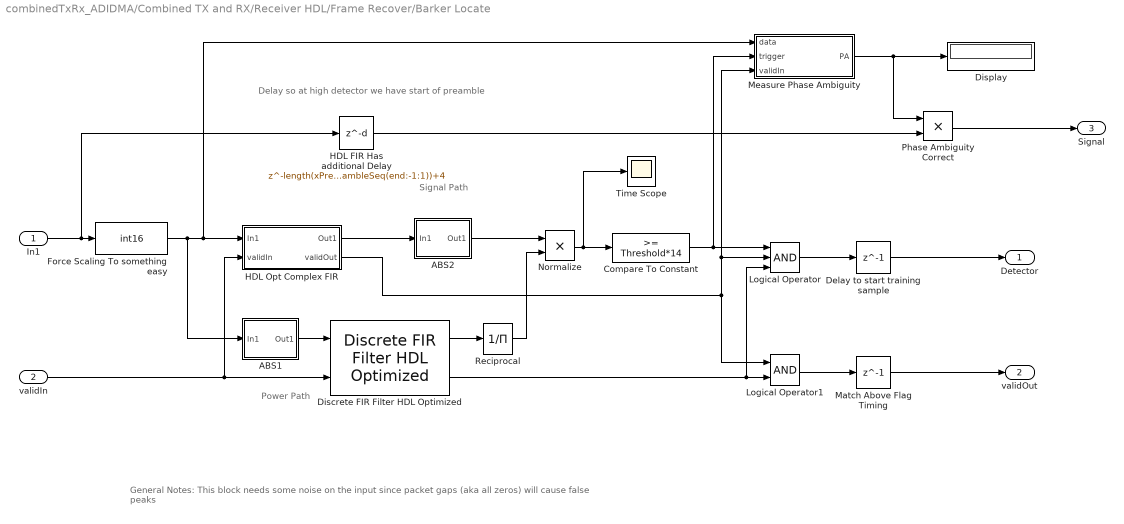
== system combinedTxRx_ADIDMA/Combined TX and RX/Receiver HDL/Frame Recover/Barker Locate ==
  note: General Notes:
      | This block needs some noise on the input since packet gaps (aka all zeros) will cause false peaks
  note: Delay so at high detector we have start of preamble
  note: Power Path
  note: Signal Path
  In1 : Inport  PortDimensions=1
  validIn : Inport  Port=2  PortDimensions=1
  ABS1 : Subsystem
  ABS2 : Subsystem
  Compare To Constant : simulink/Logic and Bit Operations/Compare To Constant  relop=>=  const=Threshold*14  OutDataTypeStr=boolean
  "Delay to start training sample " : Delay  DelayLength=1
  Discrete FIR Filter HDL Optimized : dsphdlfiltering/Discrete FIR Filter HDL Optimized  Numerator=ones(1,length(xPreambleSeq)*1)/1  Sharing=off  SharingFactor=2  SimulateUsing=Code generation  roundingMode=Floor  overflowMode=off  CoefficientsDataTypeStr=Inherit: Same word length as input  CoefficientsMin=[]  CoefficientsMax=[]  OutputDataTypeStr=fixdt(1,17,0)  OutputMin=[]  OutputMax=[]  ValidInPort=on  ReadyPort=off
      settings: SourceProductName=DSP System Toolbox  SourceProductBaseCode=DS
  Display : Display
  Force Scaling To something easy : DataTypeConversion  OutDataTypeStr=int16  SaturateOnIntegerOverflow=on
  HDL FIR Has additional Delay : Delay  DelayLength=length(xPreambleSeq(end:-1:1))+4
  HDL Opt Complex FIR : Subsystem  mask{Taps=xPreambleSeq(end:-1:1).'}
  Logical Operator : Logic  Inputs=3  AllPortsSameDT=off  OutDataTypeStr=boolean
  Logical Operator1 : Logic  AllPortsSameDT=off  OutDataTypeStr=boolean
  Match Above Flag Timing : Delay  DelayLength=1
  Measure Phase Ambiguity : Subsystem
  Normalize : Product  Inputs=**  OutDataTypeStr=int16  RndMeth=Simplest  SaturateOnIntegerOverflow=on
  Phase Ambiguity Correct : Product  OutDataTypeStr=fixdt(1,16,14)
  Reciprocal : Product  Inputs=/  SaturateOnIntegerOverflow=on  RndMeth=Zero
  Time Scope : Scope
  Detector : Outport
  validOut : Outport  Port=2
  Signal : Outport  Port=3
  wires:
  HDL Opt Complex FIR/1(Out1) -> ABS2/1(In1)
  ABS2/1(Out1) -> Normalize/1
  "Delay to start training sample "/1 -> Detector/1
  Normalize/1 -> Time Scope/1, Compare To Constant/1
  In1/1 -> HDL FIR Has additional Delay/1, Force Scaling To something easy/1
  ABS1/1(Out1) -> Discrete FIR Filter HDL Optimized/1
  Logical Operator/1 -> "Delay to start training sample "/1
  Logical Operator1/1 -> Match Above Flag Timing/1
  Measure Phase Ambiguity/1(PA) -> Display/1, Phase Ambiguity Correct/1
  validIn/1 -> HDL Opt Complex FIR/2(validIn), Discrete FIR Filter HDL Optimized/2
  Discrete FIR Filter HDL Optimized/2 -> Logical Operator1/2, Logical Operator/3
  HDL Opt Complex FIR/2(validOut) -> Logical Operator1/1, Measure Phase Ambiguity/3(validIn), Logical Operator/2
  Phase Ambiguity Correct/1 -> Signal/1
  HDL FIR Has additional Delay/1 -> Phase Ambiguity Correct/2
  Force Scaling To something easy/1 -> ABS1/1(In1), HDL Opt Complex FIR/1(In1), Measure Phase Ambiguity/1(data)
  Compare To Constant/1 -> Measure Phase Ambiguity/2(trigger), Logical Operator/1
  Discrete FIR Filter HDL Optimized/1 -> Reciprocal/1
  Reciprocal/1 -> Normalize/2
  Match Above Flag Timing/1 -> validOut/1

== system combinedTxRx_ADIDMA/Combined TX and RX/Receiver HDL/Frame Recover/Constellation Diagram After Freq Sync ==
  In1 : Inport
  Enable : EnablePort
  After Frequency Recovery : ConstellationDiagram
  wires:
  In1/1 -> After Frequency Recovery/1

== system combinedTxRx_ADIDMA/Combined TX and RX/Receiver HDL/Frame Recover/Constellation Diagram After SRRC ==
  In1 : Inport
  Enable : EnablePort
  After SRRC : ConstellationDiagram
  wires:
  In1/1 -> After SRRC/1

== system combinedTxRx_ADIDMA/Combined TX and RX/Receiver HDL/Frame Recover/Constellation Diagram After Timing ==
  In1 : Inport
  Enable : EnablePort
  After Timing Recovery : ConstellationDiagram
  wires:
  In1/1 -> After Timing Recovery/1

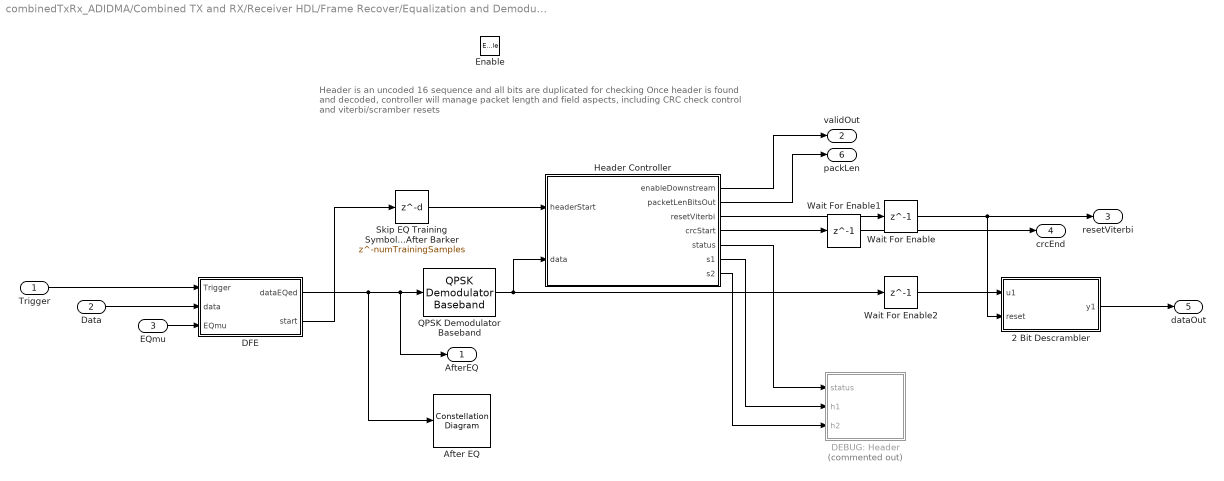
== system combinedTxRx_ADIDMA/Combined TX and RX/Receiver HDL/Frame Recover/Equalization and Demodulation ==
  note: Header is an uncoded 16 sequence and all bits are duplicated for checking
      |
      | Once header is found and decoded, controller will manage packet length and field aspects,
      | including CRC check control and viterbi/scramber resets
  Trigger : Inport
  Data : Inport  Port=2
  EQmu : Inport  Port=3
  Enable : EnablePort
  2 Bit Descrambler : Subsystem  mask{polynom=[1 1 0 1 0 1 0 1], initstate=[0 1 0 0 0 1 0]}
      mask prompts: polynom "Polynomial"; initstate "Inital State"
      mask Display: fprintf('HDL Descrambler')
  After EQ : ConstellationDiagram
  DEBUG: Header : MATLAB Function  Commented=on  TreatAsAtomicUnit=on
  DFE : Subsystem
  Header Controller : MATLAB Function  TreatAsAtomicUnit=on
  QPSK Demodulator Baseband : commdigbbndpm3/QPSK Demodulator Baseband  OutType=Bit  DecType=Hard decision  VarSource=Dialog  Variance=1  Dec=Binary  Ph=pi/4  outDtype1=boolean  outDtype2=Inherit via internal rule  derotateFactorWordLen=16  derotateFactorDataTypeStr=Inherit: Same word length as input  derotateFactorLastDataTypeStr=Inherit: Same word length as input
  Skip EQ Training Symbols After Barker : Delay  DelayLength=numTrainingSamples
  Wait For Enable : Delay  DelayLength=1
  Wait For Enable1 : Delay  DelayLength=1
  Wait For Enable2 : Delay  DelayLength=1
  AfterEQ : Outport  InitialOutput=0
  validOut : Outport  Port=2  InitialOutput=0
  resetViterbi : Outport  Port=3  InitialOutput=0
  crcEnd : Outport  Port=4  InitialOutput=0
  dataOut : Outport  Port=5  InitialOutput=0
  packLen : Outport  Port=6  InitialOutput=0
  wires:
  Skip EQ Training Symbols After Barker/1 -> Header Controller/1(headerStart)
  DFE/1(dataEQed) -> AfterEQ/1, QPSK Demodulator Baseband/1, After EQ/1
  QPSK Demodulator Baseband/1 -> Header Controller/2(data), Wait For Enable2/1
  Header Controller/1(enableDownstream) -> validOut/1
  Header Controller/4(crcStart) -> Wait For Enable1/1
  Header Controller/3(resetViterbi) -> Wait For Enable/1
  Header Controller/2(packetLenBitsOut) -> packLen/1
  Wait For Enable/1 -> 2 Bit Descrambler/2(reset), resetViterbi/1
  Wait For Enable1/1 -> crcEnd/1
  Wait For Enable2/1 -> 2 Bit Descrambler/1(u1)
  2 Bit Descrambler/1(y1) -> dataOut/1
  Trigger/1 -> DFE/1(Trigger)
  Data/1 -> DFE/2(data)
  DFE/2(start) -> Skip EQ Training Symbols After Barker/1
  EQmu/1 -> DFE/3(EQmu)
  Header Controller/5(status) -> DEBUG: Header/1(status)
  Header Controller/6(s1) -> DEBUG: Header/2(h1)
  Header Controller/7(s2) -> DEBUG: Header/3(h2)

== system combinedTxRx_ADIDMA/Combined TX and RX/Receiver HDL/Frame Recover/Frequency Recovery ==
  note: Decrease Loop bandwidth to reduce phase noise,
      | but worse pull-in range
      | -0.1 30kHz pull-in
      | -0.01 5kHz pull-in
  note: Max Phase Lock Delay= 1.3/(NormLoopBandwidth*SampleRate)
  note: Frequency Lock Delay = SampleRate*4*NormalizedPullInRange^2)/ (SampleRate*NormLoopBandwidth)^3;
  note: Pull in range (Hz) = 2*pi*sqrt(2)*DampingFactor*NormLoopBandwidth*SampleRate
  dataIn : Inport
  validIn : Inport  Port=2
  LoopBW : Inport  Port=3
  Enable : EnablePort
  Delay : Delay  DelayLength=1
  Loop Filter : Subsystem  Commented=on  mask{BnTs=0.1, zeta=4*1/sqrt(2), N=1}
      mask prompts: BnTs "Normalized Loop Bandwidth"; zeta "Damping Factor"; N "Number of Samples/Symbol"
      mask init:
      | % See C.57 to C.61 in Michael Rice's "Digital Communications 
      | % - A Discrete-Time Approach" for details
      | 
      | %theta = BnTs/(zeta+0.25/zeta);  %0.0385
      | %d = 1 + 2*zeta*theta + theta*theta; %1.1938
      | %K1 = zeta*theta/d; %0.0805
      | %K2 = theta*theta/(d*2); %6.1958e-04
      | 
      | %%
      | DampingFactor = zeta;
      | samplesPerSymbol = N;
      | NormalizedLoopBandwidth = BnTs;
      | %
      | PhaseRecoveryLoopBandwidth = NormalizedLoopBandwidth*samplesPerSymbol;
      |  
      | PhaseRecoveryGain = samplesPerSymbol;
      |  
      | PhaseErrorDetectorGain = 1;
      | 
      | 
      | theta = PhaseRecoveryLoopBandwidth/...
      |     ((DampingFactor + 0.25/DampingFactor)*samplesPerSymbol);
      |  
      | d = 1 + 2*DampingFactor*theta + theta*theta;
      |  
      | % K1
      | K1 = (4*DampingFactor*theta/d)/...
      |     (PhaseErrorDetectorGain*PhaseRecoveryGain);
      | % K2
      | K2 = (4/samplesPerSymbol*theta*theta/d)/...
      |     (PhaseErrorDetectorGain*PhaseRecoveryGain);
      mask Display: disp('Loop Filter')
  Loop Filter Configurable : Subsystem
      mask Display: disp('Loop Filter')
  PED : MATLAB Function  TreatAsAtomicUnit=on
  Phase Shift FP : Subsystem
  State Control : StateControl  StateControl=Synchronous
  dataOut : Outport
  validOut : Outport  Port=2
  wires:
  Delay/1 -> PED/1(In), dataOut/1
  PED/1(e) -> Loop Filter Configurable/1(e)
  Loop Filter Configurable/1(v) -> Phase Shift FP/2(Phi)
  dataIn/1 -> Phase Shift FP/1(In1)
  Phase Shift FP/1(Out1) -> Delay/1
  validIn/1 -> validOut/1
  LoopBW/1 -> Loop Filter Configurable/2(LoopBW)

== system combinedTxRx_ADIDMA/Combined TX and RX/Receiver HDL/Frame Recover/Gardner Timing Recovery ==
  In1 : Inport
  Enable : EnablePort
  Delay : Delay  DelayLength=1
  Delay1 : Delay  DelayLength=1
  Delay2 : Delay  DelayLength=6
  Gardner TED Blocks : Subsystem
  InterpControl_Blocks1 : Subsystem
  Interpolator : Subsystem
  LoopFilter1 : Subsystem  mask{zeta=sqrt(2), BnTs=0.01, Kp=2.7}
      mask prompts: zeta "DampingFactor"; BnTs "NormalizedLoopBandwidth"; Kp "DetectionGain"
      mask init:
      | K0 = -1;
      | SPS = 4;
      | theta = BnTs/SPS/(zeta + 0.25/zeta);
      | d  = (1 + 2*zeta*theta + theta^2) * K0 * Kp;
      | ProportionalGain = (4*zeta*theta) /d;
      | IntegratorGain   = (4*theta*theta)/d;
  State Control : StateControl  StateControl=Synchronous
  Out1 : Outport  InitialOutput=0
  strobe : Outport  Port=2  InitialOutput=false
  wires:
  In1/1 -> Delay2/1
  Delay1/1 -> Gardner TED Blocks/2(strobe), strobe/1
  Delay/1 -> Interpolator/2(mu)
  Interpolator/1(Out1) -> Gardner TED Blocks/1(data), Out1/1
  Gardner TED Blocks/1(e) -> LoopFilter1/1(e)
  InterpControl_Blocks1/1(strobe) -> Delay1/1
  InterpControl_Blocks1/2(mu) -> Delay/1
  LoopFilter1/1(v) -> InterpControl_Blocks1/1(e)
  Delay2/1 -> Interpolator/1(In1)

== system combinedTxRx_ADIDMA/Combined TX and RX/Transmitter HDL/Transmitter HDL/DMA Interface ==
  byteIn : Inport
  validIn : Inport  Port=2
  EOF : Inport  Port=3
  Align with data : Delay  DelayLength=1
  DMA Control : MATLAB Function  TreatAsAtomicUnit=on
  validOut : Outport
  bit : Outport  Port=2
  payloadLength : Outport  Port=3  OutDataTypeStr=uint16
  startOut : Outport  Port=4
  readyForMore : Outport  Port=5
  wires:
  byteIn/1 -> DMA Control/1(byteIn)
  DMA Control/1(bitOut) -> bit/1
  DMA Control/5(readyForInput) -> readyForMore/1
  DMA Control/4(payloadLength) -> payloadLength/1
  DMA Control/2(validOut) -> validOut/1
  validIn/1 -> DMA Control/2(validIn)
  Align with data/1 -> startOut/1
  DMA Control/3(startOut) -> Align with data/1
  EOF/1 -> DMA Control/3(EOF)

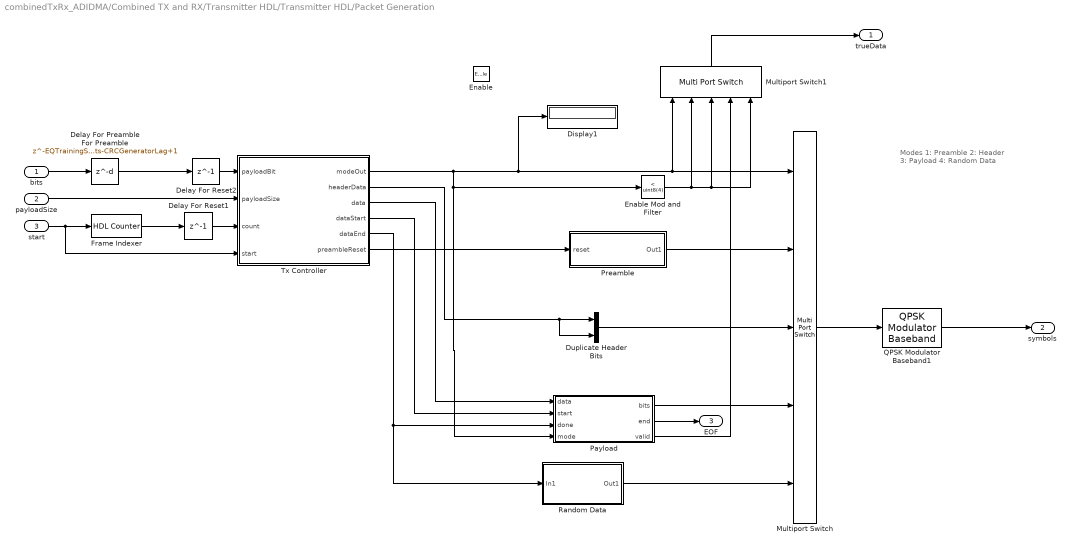
== system combinedTxRx_ADIDMA/Combined TX and RX/Transmitter HDL/Transmitter HDL/Packet Generation ==
  note: Modes
      | 	1: Preamble
      | 	2: Header
      | 	3: Payload
      | 	4: Random Data
  bits : Inport  OutDataTypeStr=boolean
  payloadSize : Inport  Port=2
  start : Inport  Port=3
  Enable : EnablePort
  Delay For Preamble For Preamble : Delay  DelayLength=EQTrainingSymbols+AGCBarkerSymbols+numHeaderBits-CRCGeneratorLag+1  InitialCondition=false
  Delay For Reset1 : Delay  DelayLength=1
  Delay For Reset2 : Delay  DelayLength=1  InitialCondition=false
  Display1 : Display
  Duplicate Header Bits : Concatenate
  Enable Mod and Filter : simulink/Logic and Bit Operations/Compare To Constant  relop=<  const=uint8(4)  OutDataTypeStr=boolean
  Frame Indexer : hdlsllib/Sources/HDL Counter  CountType=Count limited  CountInit=0  CountStep=1  CountMax=2^16+EQTrainingSymbols+AGCBarkerSymbols+numHeaderBits  CountFromType=Specify  CountFrom=0  CountResetPort=on  CountLoadPort=off  CountEnbPort=off  CountDirPort=off  CountDataType=Unsigned  CountWordLen=32  CountFracLen=0  CountSampTime=1
      settings: SourceProductBaseCode=HD
  Multiport Switch : MultiPortSwitch  Inputs=4
  Multiport Switch1 : MultiPortSwitch  Inputs=4
  Payload : Subsystem
  Preamble : Subsystem
  QPSK Modulator Baseband1 : commdigbbndpm3/QPSK Modulator Baseband  InType=Bit  Enc=Binary  Ph=pi/4  outDtype=Fixed-point  outWordLen=16  outUDDataType=sfix(16)  outFracLenMode=User-defined  outFracLen=15  outDataTypeStr=fixdt(1,16,15)  outLastDataTypeStr=fixdt(1,16,15)
  Random Data : Subsystem
  Tx Controller : MATLAB Function  TreatAsAtomicUnit=on
  trueData : Outport  InitialOutput=0
  symbols : Outport  Port=2  InitialOutput=complex(0)
  EOF : Outport  Port=3  OutDataTypeStr=boolean  InitialOutput=0
  wires:
  Tx Controller/2(headerData) -> Duplicate Header Bits/2, Duplicate Header Bits/1
  Random Data/1(Out1) -> Multiport Switch/5
  Enable Mod and Filter/1 -> Multiport Switch1/5, Multiport Switch1/3, Multiport Switch1/2
  Tx Controller/3(data) -> Payload/1(data)
  Tx Controller/4(dataStart) -> Payload/2(start)
  Delay For Preamble For Preamble/1 -> Delay For Reset2/1
  start/1 -> Tx Controller/4(start), Frame Indexer/1
  Preamble/1(Out1) -> Multiport Switch/2
  bits/1 -> Delay For Preamble For Preamble/1
  QPSK Modulator Baseband1/1 -> symbols/1
  Multiport Switch1/1 -> trueData/1
  Delay For Reset1/1 -> Tx Controller/3(count)
  Multiport Switch/1 -> QPSK Modulator Baseband1/1
  Tx Controller/5(dataEnd) -> Payload/3(done), Random Data/1(In1)
  Payload/1(bits) -> Multiport Switch/4
  Duplicate Header Bits/1 -> Multiport Switch/3
  Frame Indexer/1 -> Delay For Reset1/1
  Payload/3(valid) -> Multiport Switch1/4
  Payload/2(end) -> EOF/1
  payloadSize/1 -> Tx Controller/2(payloadSize)
  Tx Controller/1(modeOut) -> Display1/1, Multiport Switch/1, Multiport Switch1/1, Payload/4(mode), Enable Mod and Filter/1
  Tx Controller/6(preambleReset) -> Preamble/1(reset)
  Delay For Reset2/1 -> Tx Controller/1(payloadBit)

== system combinedTxRx_ADIDMA/Combined TX and RX/Receiver HDL/CRC Check and DMA Pack/DMA Interface/Convert Payload Length To Bytes ==
  In1 : Inport
  Constant : Constant  Value=uint16(32-1)  SampleTime=-1
  Convert To Bytes From Bits : ArithShift  BitShiftNumber=3  BitShiftDirection=Right
  Convert To Uncoded : ArithShift  BitShiftNumber=1  BitShiftDirection=Right
  Data Type Conversion : DataTypeConversion  OutDataTypeStr=uint16
  Remove CRC Length : Sum  Inputs=+-  AccumDataTypeStr=uint16
  Out1 : Outport
  wires:
  In1/1 -> Convert To Uncoded/1
  Remove CRC Length/1 -> Convert To Bytes From Bits/1
  Convert To Uncoded/1 -> Remove CRC Length/1
  Convert To Bytes From Bits/1 -> Data Type Conversion/1
  Constant/1 -> Remove CRC Length/2
  Data Type Conversion/1 -> Out1/1

== system combinedTxRx_ADIDMA/Combined TX and RX/Receiver HDL/Frame Recover/Barker Locate/ABS1 ==
  In1 : Inport
  Add : Sum
  Complex to Real-Imag : ComplexToRealImag
  Product : Product  OutDataTypeStr=int16
  Product1 : Product  OutDataTypeStr=int16
  Out1 : Outport
  wires:
  In1/1 -> Complex to Real-Imag/1
  Complex to Real-Imag/2 -> Product1/2, Product1/1
  Complex to Real-Imag/1 -> Product/1, Product/2
  Product/1 -> Add/1
  Product1/1 -> Add/2
  Add/1 -> Out1/1

== system combinedTxRx_ADIDMA/Combined TX and RX/Receiver HDL/Frame Recover/Barker Locate/ABS2 ==
  In1 : Inport
  Add : Sum  SaturateOnIntegerOverflow=on
  Complex to Real-Imag : ComplexToRealImag
  Product : Product  OutDataTypeStr=int16
  Product1 : Product  OutDataTypeStr=int16
  Out1 : Outport
  wires:
  In1/1 -> Complex to Real-Imag/1
  Complex to Real-Imag/2 -> Product1/2, Product1/1
  Complex to Real-Imag/1 -> Product/1, Product/2
  Product/1 -> Add/1
  Product1/1 -> Add/2
  Add/1 -> Out1/1

== system combinedTxRx_ADIDMA/Combined TX and RX/Receiver HDL/Frame Recover/Barker Locate/HDL Opt Complex FIR ==
  In1 : Inport
  validIn : Inport  Port=2
  Add : Sum  AccumDataTypeStr=fixdt(1,16,0)
  Discrete FIR Filter HDL Optimized : dsphdlfiltering/Discrete FIR Filter HDL Optimized  Numerator=real(Taps)  Sharing=off  SharingFactor=2  SimulateUsing=Code generation  roundingMode=Floor  overflowMode=off  CoefficientsDataTypeStr=Inherit: Same word length as input  CoefficientsMin=[]  CoefficientsMax=[]  OutputDataTypeStr=fixdt(1,15,0)  OutputMin=[]  OutputMax=[]  ValidInPort=on  ReadyPort=off
      settings: SourceProductName=DSP System Toolbox  SourceProductBaseCode=DS
  Discrete FIR Filter HDL Optimized1 : dsphdlfiltering/Discrete FIR Filter HDL Optimized  Numerator=imag(Taps)  Sharing=off  SharingFactor=2  SimulateUsing=Code generation  roundingMode=Floor  overflowMode=off  CoefficientsDataTypeStr=Inherit: Same word length as input  CoefficientsMin=[]  CoefficientsMax=[]  OutputDataTypeStr=fixdt(1,15,0)  OutputMin=[]  OutputMax=[]  ValidInPort=on  ReadyPort=off
      settings: SourceProductName=DSP System Toolbox  SourceProductBaseCode=DS
  Logical Operator : Logic  AllPortsSameDT=off  OutDataTypeStr=boolean
  Out1 : Outport
  validOut : Outport  Port=2
  wires:
  In1/1 -> Discrete FIR Filter HDL Optimized1/1, Discrete FIR Filter HDL Optimized/1
  Discrete FIR Filter HDL Optimized/1 -> Add/1
  Add/1 -> Out1/1
  Logical Operator/1 -> validOut/1
  Discrete FIR Filter HDL Optimized/2 -> Logical Operator/1
  Discrete FIR Filter HDL Optimized1/2 -> Logical Operator/2
  Discrete FIR Filter HDL Optimized1/1 -> Add/2
  validIn/1 -> Discrete FIR Filter HDL Optimized1/2, Discrete FIR Filter HDL Optimized/2

== system combinedTxRx_ADIDMA/Combined TX and RX/Receiver HDL/Frame Recover/Barker Locate/Measure Phase Ambiguity ==
  data : Inport  OutDataTypeStr=int16
  trigger : Inport  Port=2
  validIn : Inport  Port=3
  Find Max and Set Output Shift : Subsystem
  HDL Opt Complex FIR4 : Subsystem  mask{Taps=xPreambleSeq(end:-1:1).'}
  HDL Opt Complex FIR5 : Subsystem  mask{Taps=exp(-j*pi/2).*xPreambleSeq(end:-1:1).'}
  HDL Opt Complex FIR6 : Subsystem  mask{Taps=exp(-j*pi).*xPreambleSeq(end:-1:1).'}
  HDL Opt Complex FIR7 : Subsystem  mask{Taps=exp(-j*pi*3/2).*xPreambleSeq(end:-1:1).'}
  Logical Operator : Logic  Inputs=5  AllPortsSameDT=off  OutDataTypeStr=boolean
  PA : Outport  InitialOutput=0
  wires:
  data/1 -> HDL Opt Complex FIR4/1(In1), HDL Opt Complex FIR5/1(In1), HDL Opt Complex FIR7/1(In1), HDL Opt Complex FIR6/1(In1)
  HDL Opt Complex FIR4/1(Out1) -> Find Max and Set Output Shift/1(In1)
  HDL Opt Complex FIR5/1(Out1) -> Find Max and Set Output Shift/2(In2)
  HDL Opt Complex FIR6/1(Out1) -> Find Max and Set Output Shift/3(In4)
  HDL Opt Complex FIR7/1(Out1) -> Find Max and Set Output Shift/4(In5)
  Find Max and Set Output Shift/1(Out1) -> PA/1
  validIn/1 -> HDL Opt Complex FIR4/2(validIn), HDL Opt Complex FIR5/2(validIn), HDL Opt Complex FIR7/2(validIn), HDL Opt Complex FIR6/2(validIn)
  HDL Opt Complex FIR4/2(validOut) -> Logical Operator/1
  HDL Opt Complex FIR5/2(validOut) -> Logical Operator/2
  HDL Opt Complex FIR6/2(validOut) -> Logical Operator/3
  HDL Opt Complex FIR7/2(validOut) -> Logical Operator/4
  Logical Operator/1 -> Find Max and Set Output Shift/Enable
  trigger/1 -> Logical Operator/5

== system combinedTxRx_ADIDMA/Combined TX and RX/Receiver HDL/Frame Recover/Equalization and Demodulation/2 Bit Descrambler ==
  note: This is a special Descrambler which can process 2 bits at a time
  u1 : Inport
  reset : Inport  Port=2
  Demux1 : Demux  Outputs=2
  MATLAB Function : MATLAB Function  TreatAsAtomicUnit=on
  Mux : Mux  Inputs=2
  Selector1 : Selector  IndexOptions=Index vector (dialog)  Indices=find(polynom(2:end))  OutputSizes=1
  Selector2 : Selector  IndexOptions=Index vector (dialog)  Indices=find(polynom(2:end))  OutputSizes=1
  input_xor1 : Logic  Operator=XOR  IconShape=distinctive  AllPortsSameDT=off  OutDataTypeStr=boolean
  input_xor2 : Logic  Operator=XOR  IconShape=distinctive  AllPortsSameDT=off  OutDataTypeStr=boolean
  state_xor1 : Logic  Operator=XOR  Inputs=1  IconShape=distinctive  AllPortsSameDT=off  OutDataTypeStr=boolean
  state_xor2 : Logic  Operator=XOR  Inputs=1  IconShape=distinctive  AllPortsSameDT=off  OutDataTypeStr=boolean
  y1 : Outport  InitialOutput=0
  wires:
  u1/1 -> Demux1/1, MATLAB Function/1(bits)
  reset/1 -> MATLAB Function/2(reset)
  MATLAB Function/1(bufferA) -> Selector1/1
  MATLAB Function/2(bufferB) -> Selector2/1
  Mux/1 -> y1/1
  state_xor1/1 -> input_xor1/1
  state_xor2/1 -> input_xor2/1
  input_xor2/1 -> Mux/2
  input_xor1/1 -> Mux/1
  Selector1/1 -> state_xor1/1
  Selector2/1 -> state_xor2/1
  Demux1/1 -> input_xor1/2
  Demux1/2 -> input_xor2/2  "data_in"
